simulink model "ekf2sfb"  (R2014a)
settings: Solver=FixedStepDiscrete  StartTime=0.0  StopTime=100.0  RelTol=1e-3
values from neighbouring files (symbols this model uses):
  T = block.DialogPrm(6).Data    [sfall2.m]    (also in sysall.m = 0.05)
undefined symbols (not defined in the file or in its folder): Q, R
libraries: simulink x3
settings Model: Creator=gcampa  LastModifiedBy=gcampa
settings DataIOCC: SignalLoggingSaveFormat=ModelDataLogs  SaveOutput=off  SignalLogging=off  DSMLogging=off  SaveTime=off
settings OptimizationCC: ExpressionDepthLimit=2147483647  InitFltsAndDblsToZero=on
settings DebuggingCC: SaveWithParameterizedLinksMsg=none  UnderspecifiedInitializationDetection=Classic  SignalResolutionControl=TryResolveAllWithWarning  MultiTaskDSMMsg=warning  MultiTaskCondExecSysMsg=none  FcnCallInpInsideContextMsg=UseLocalSettings  StateNameClashWarn=warning
settings SFSimCC: SimParseCustomCode=off
settings RTWCC: IncludeERTFirstTime=on  RTWCompilerOptimization=On
settings GRTTargetCC: TargetFcnLib=ansi_tfl_tmw.mat  CombineOutputUpdateFcns=off  GRTInterface=on

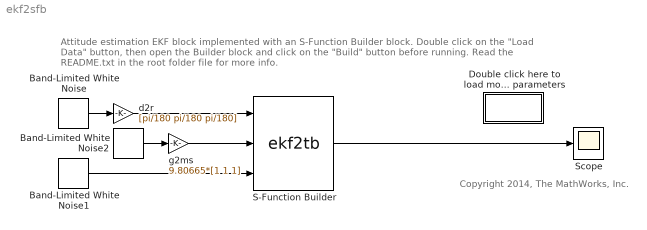
== system ekf2sfb ==
  note: Attitude estimation EKF block implemented with an S-Function Builder block.
      | Double click on the "Load Data" button, then open the Builder block and click on the "Build" button before running.
      | Read the README.txt in the root folder file for more info.
  note: Copyright 2014, The MathWorks, Inc.
  Band-Limited White Noise : simulink/Sources/Band-Limited White Noise  Cov=0.1*[1 1 1]  Ts=T  seed=[1 2 3]
  Band-Limited White Noise1 : simulink/Sources/Band-Limited White Noise  Cov=0.1*[1 1 1]  Ts=T  seed=[7 8 9]
  Band-Limited White Noise2 : simulink/Sources/Band-Limited White Noise  Cov=0.1*[1 1 1]  Ts=T  seed=[4 5 6]
  Double click here to load model and parameters : Subsystem
      settings: OpenFcn=|
      | V_0= 21.44176640107837;
      | phi_0=0.16673723163960;
      | theta_0=0.38249284705297;
      | psi_0=-3.10672050096899;
      | 
      | Q= [1.1339e-006     0               0
      |     0               3.1232e-006     0
      |     0               0               2.9009e-006];
      | 
      | R= [0.3368          0               0
      |     0               0.092           0
      |     0               0               0];
      | 
      | T=0.05;
      mask Display: disp('Load\nData')
  S-Function Builder : S-Function  InitFcn=try, set_param(gcb,'FunctionName','ekf2tb'), end  FunctionName=ekf2tb  Parameters=Q(1:2,1:2),R(1:2,1:2),1e-5  SFunctionModules=ekf2tb_wrapper  EnableBusSupport=off  mask(S-Function Builder){}
      mask init:
      | val = [[.9  0.75 0.75 1 1 .9 .9 1]',[1 1 0.75 0.75 .9 .9 1 .9]'];try , sys = get_param(gcb,'SfunBuilderFcnName');if isempty(sys), sys = get_param(gcb,'FunctionName'); end,catch, sys = get_param(gcb,'FunctionName'); end
      settings: CopyFcn=set_param(gcbh,'LinkStatus','none')  PreSaveFcn=try, set_param(gcb,'FunctionName','ekf2tb'), end  OpenFcn=sfunctionwizard(gcbh)
      mask Display: plot(val(:,1),val(:,2)),disp(sys), port_label('input',1,'pqr'), port_label('input',2,'a_b'), port_label('input',3,'v_e'), port_label('output',1,'rpy')
  Scope : Scope
      settings: TimeRange=100  YMin=-4  YMax=4
  d2r : Gain  Gain=[pi/180 pi/180 pi/180]  SaturateOnIntegerOverflow=on  OutDataTypeStr=Inherit: Same as input  ParamDataTypeStr=Inherit: Same as input
  g2ms : Gain  Gain=9.80665*[1 1 1]  SaturateOnIntegerOverflow=on  OutDataTypeStr=Inherit: Same as input  ParamDataTypeStr=Inherit: Same as input
  wires:
  Band-Limited White Noise/1 -> d2r/1
  Band-Limited White Noise1/1 -> S-Function Builder/3
  Band-Limited White Noise2/1 -> g2ms/1
  d2r/1 -> S-Function Builder/1
  g2ms/1 -> S-Function Builder/2
  S-Function Builder/1 -> Scope/1

== system ekf2sfb/Double click here to load model and parameters ==
